simulink model "FourActuatorAWD"  (R2026b)
settings: Solver=VariableStepAuto
settings Model: Creator=The MathWorks, Inc.  LastModifiedBy=The MathWorks, Inc.
settings OptimizationCC: ReuseModelBlockBuffer=off

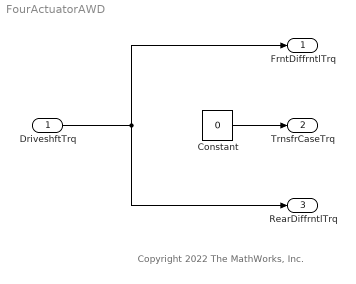
== system FourActuatorAWD ==
  note: Copyright 2022 The MathWorks, Inc.
  DriveshftTrq : Inport
  Constant : Constant  Value=0  SampleTime=-1
  FrntDiffrntlTrq : Outport
  TrnsfrCaseTrq : Outport  Port=2
  RearDiffrntlTrq : Outport  Port=3
  wires:
  DriveshftTrq/1 -> RearDiffrntlTrq/1, FrntDiffrntlTrq/1
  Constant/1 -> TrnsfrCaseTrq/1
